simulink model "TestApp"  (R2014a)
settings: Solver=ode45  StartTime=0.0  StopTime=1  RelTol=1e-3
libraries: simulink x6, arduinolib x4
settings Model: Creator=beaverl  LastModifiedBy=beaverl

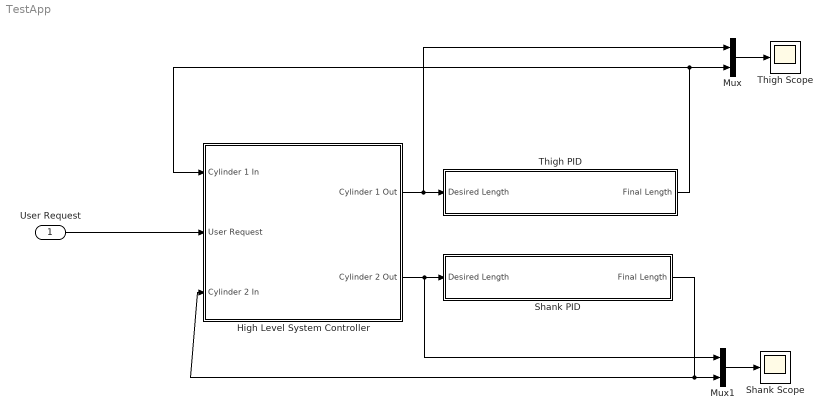
== system TestApp ==
  User Request : Inport
  High Level System Controller : Subsystem
  Mux : Mux  Inputs=2
  Mux1 : Mux  Inputs=2
  Shank PID : Subsystem
  Shank Scope : Scope
      settings: TimeRange=1  YMin=0  YMax=10
  Thigh PID : Subsystem
  Thigh Scope : Scope
      settings: TimeRange=1  YMin=0  YMax=10
  wires:
  Thigh PID/1(Final Length) -> High Level System Controller/1(Cylinder 1 In), Mux/2
  High Level System Controller/1(Cylinder 1 Out) -> Mux/1, Thigh PID/1(Desired Length)
  High Level System Controller/2(Cylinder 2 Out) -> Shank PID/1(Desired Length), Mux1/1
  Shank PID/1(Final Length) -> Mux1/2, High Level System Controller/3(Cylinder 2 In)
  Mux/1 -> Thigh Scope/1
  Mux1/1 -> Shank Scope/1
  User Request/1 -> High Level System Controller/2(User Request)

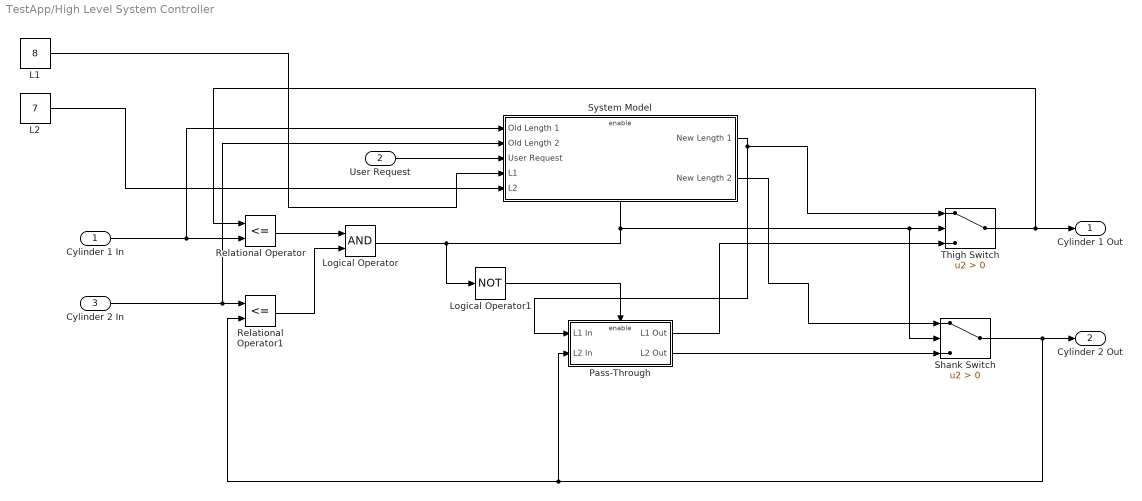
== system TestApp/High Level System Controller ==
  Cylinder 1 In : Inport
  User Request : Inport  Port=2
  Cylinder 2 In : Inport  Port=3
  L1 : Constant  Value=8
  L2 : Constant  Value=7
  Logical Operator : Logic  AllPortsSameDT=off  OutDataTypeStr=boolean
  Logical Operator1 : Logic  Operator=NOT  AllPortsSameDT=off  OutDataTypeStr=boolean
  Pass-Through : Subsystem  TreatAsAtomicUnit=on
  Relational Operator : RelationalOperator  Operator=<=  OutDataTypeStr=boolean
  Relational Operator1 : RelationalOperator  Operator=<=  OutDataTypeStr=boolean
  Shank Switch : Switch  Criteria=u2 > Threshold
  System Model : Subsystem
  Thigh Switch : Switch  Criteria=u2 > Threshold
  Cylinder 1 Out : Outport
  Cylinder 2 Out : Outport  Port=2
  wires:
  Cylinder 2 In/1 -> System Model/2(Old Length 2), Relational Operator1/1
  Cylinder 1 In/1 -> System Model/1(Old Length 1), Relational Operator/2
  System Model/1(New Length 1) -> Pass-Through/1(L1 In), Thigh Switch/1
  System Model/2(New Length 2) -> Shank Switch/1
  Relational Operator/1 -> Logical Operator/1
  Relational Operator1/1 -> Logical Operator/2
  Logical Operator/1 -> Logical Operator1/1, Shank Switch/2, Thigh Switch/2, System Model/Enable
  Logical Operator1/1 -> Pass-Through/Enable
  User Request/1 -> System Model/3(User Request)
  Thigh Switch/1 -> Relational Operator/1, Cylinder 1 Out/1
  Pass-Through/1(L1 Out) -> Thigh Switch/3
  Pass-Through/2(L2 Out) -> Shank Switch/3
  Shank Switch/1 -> Pass-Through/2(L2 In), Relational Operator1/2, Cylinder 2 Out/1
  L1/1 -> System Model/4(L1)
  L2/1 -> System Model/5(L2)

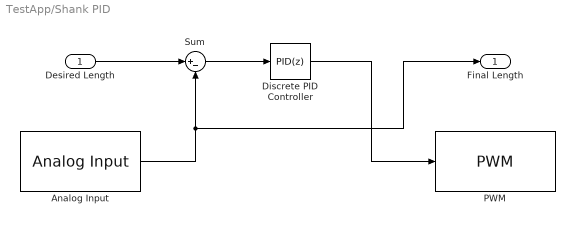
== system TestApp/Shank PID ==
  Desired Length : Inport
  Analog Input : arduinolib/Analog Input  pinNumber=6  sampleTime=-1
  Discrete PID Controller : simulink/Continuous/PID Controller  Controller=PID  TimeDomain=Discrete-time  SampleTime=-1  IntegratorMethod=Forward Euler  FilterMethod=Forward Euler  Form=Parallel  P=25  I=0.78  D=0  N=100  InitialConditionSource=internal  InitialConditionForIntegrator=0  InitialConditionForFilter=0  ExternalReset=none  LimitOutput=off  UpperSaturationLimit=inf  LowerSaturationLimit=-inf  LinearizeAsGain=off  AntiWindupMode=none  Kb=1  TrackingMode=off  Kt=1  PParamMin=[]  PParamMax=[]  IParamMin=[]  IParamMax=[]  DParamMin=[]  DParamMax=[]  NParamMin=[]  NParamMax=[]  KbParamMin=[]  KbParamMax=[]  KtParamMin=[]  KtParamMax=[]  POutMin=[]  POutMax=[]  IOutMin=[]  IOutMax=[]  DOutMin=[]  DOutMax=[]  NOutMin=[]  NOutMax=[]  KbOutMin=[]  KbOutMax=[]  KtOutMin=[]  KtOutMax=[]  IntegratorOutMin=[]  IntegratorOutMax=[]  FilterOutMin=[]  FilterOutMax=[]  SumOutMin=[]  SumOutMax=[]  SumI1OutMin=[]  SumI1OutMax=[]  SumI2OutMin=[]  SumI2OutMax=[]  SumI3OutMin=[]  SumI3OutMax=[]  SumDOutMin=[]  SumDOutMax=[]  SaturationOutMin=[]  SaturationOutMax=[]  IntegratorContinuousStateAttributes=''  IntegratorStateMustResolveToSignalObject=off  IntegratorRTWStateStorageClass=Auto  FilterContinuousStateAttributes=''  FilterStateMustResolveToSignalObject=off  FilterRTWStateStorageClass=Auto
  PWM : arduinolib/PWM  pinNumber=7
  Sum : Sum  Inputs=|+-
  Final Length : Outport
  wires:
  Desired Length/1 -> Sum/1
  Analog Input/1 -> Final Length/1, Sum/2
  Sum/1 -> Discrete PID Controller/1
  Discrete PID Controller/1 -> PWM/1

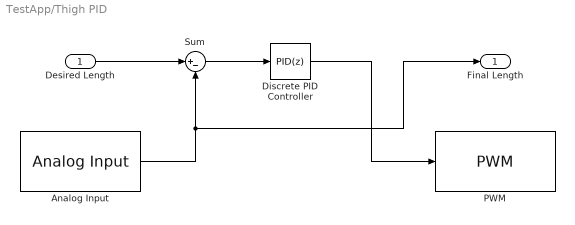
== system TestApp/Thigh PID ==
  Desired Length : Inport
  Analog Input : arduinolib/Analog Input  pinNumber=4  sampleTime=-1
  Discrete PID Controller : simulink/Continuous/PID Controller  Controller=PID  TimeDomain=Discrete-time  SampleTime=-1  IntegratorMethod=Forward Euler  FilterMethod=Forward Euler  Form=Parallel  P=25  I=0.78  D=0  N=100  InitialConditionSource=internal  InitialConditionForIntegrator=0  InitialConditionForFilter=0  ExternalReset=none  LimitOutput=off  UpperSaturationLimit=inf  LowerSaturationLimit=-inf  LinearizeAsGain=off  AntiWindupMode=none  Kb=1  TrackingMode=off  Kt=1  PParamMin=[]  PParamMax=[]  IParamMin=[]  IParamMax=[]  DParamMin=[]  DParamMax=[]  NParamMin=[]  NParamMax=[]  KbParamMin=[]  KbParamMax=[]  KtParamMin=[]  KtParamMax=[]  POutMin=[]  POutMax=[]  IOutMin=[]  IOutMax=[]  DOutMin=[]  DOutMax=[]  NOutMin=[]  NOutMax=[]  KbOutMin=[]  KbOutMax=[]  KtOutMin=[]  KtOutMax=[]  IntegratorOutMin=[]  IntegratorOutMax=[]  FilterOutMin=[]  FilterOutMax=[]  SumOutMin=[]  SumOutMax=[]  SumI1OutMin=[]  SumI1OutMax=[]  SumI2OutMin=[]  SumI2OutMax=[]  SumI3OutMin=[]  SumI3OutMax=[]  SumDOutMin=[]  SumDOutMax=[]  SaturationOutMin=[]  SaturationOutMax=[]  IntegratorContinuousStateAttributes=''  IntegratorStateMustResolveToSignalObject=off  IntegratorRTWStateStorageClass=Auto  FilterContinuousStateAttributes=''  FilterStateMustResolveToSignalObject=off  FilterRTWStateStorageClass=Auto
  PWM : arduinolib/PWM  pinNumber=5
  Sum : Sum  Inputs=|+-
  Final Length : Outport
  wires:
  Desired Length/1 -> Sum/1
  Analog Input/1 -> Final Length/1, Sum/2
  Sum/1 -> Discrete PID Controller/1
  Discrete PID Controller/1 -> PWM/1

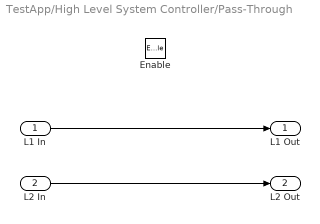
== system TestApp/High Level System Controller/Pass-Through ==
  L1 In : Inport
  L2 In : Inport  Port=2
  Enable : EnablePort
  L1 Out : Outport
  L2 Out : Outport  Port=2
  wires:
  L1 In/1 -> L1 Out/1
  L2 In/1 -> L2 Out/1

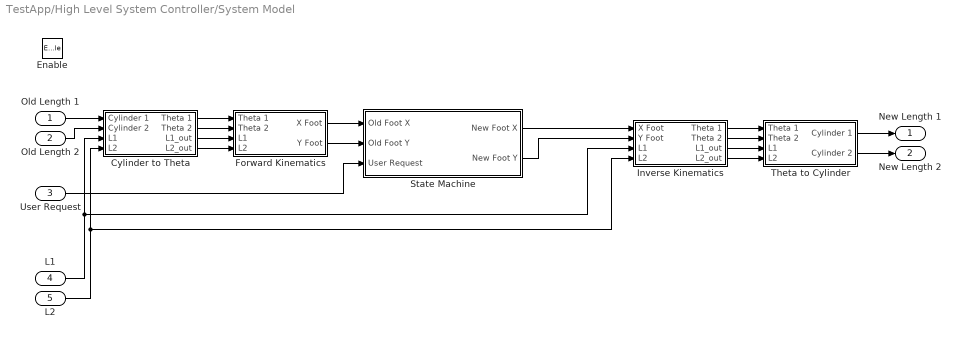
== system TestApp/High Level System Controller/System Model ==
  Old Length 1 : Inport
  Old Length 2 : Inport  Port=2
  User Request : Inport  Port=3
  L1 : Inport  Port=4
  L2 : Inport  Port=5
  Enable : EnablePort
  Cylinder to Theta : Subsystem
  Forward Kinematics : Subsystem
  Inverse Kinematics : Subsystem
  State Machine : Subsystem
  Theta to Cylinder : Subsystem
  New Length 1 : Outport
  New Length 2 : Outport  Port=2
  wires:
  Old Length 1/1 -> Cylinder to Theta/1(Cylinder 1)
  Old Length 2/1 -> Cylinder to Theta/2(Cylinder 2)
  Theta to Cylinder/2(Cylinder 2) -> New Length 2/1
  Theta to Cylinder/1(Cylinder 1) -> New Length 1/1
  Cylinder to Theta/1(Theta 1) -> Forward Kinematics/1(Theta 1)
  Cylinder to Theta/2(Theta 2) -> Forward Kinematics/2(Theta 2)
  Forward Kinematics/1(X Foot) -> State Machine/1(Old Foot X)
  Forward Kinematics/2(Y Foot) -> State Machine/2(Old Foot Y)
  State Machine/1(New Foot X) -> Inverse Kinematics/1(X Foot)
  State Machine/2(New Foot Y) -> Inverse Kinematics/2(Y Foot)
  Inverse Kinematics/1(Theta 1) -> Theta to Cylinder/1(Theta 1)
  Inverse Kinematics/2(Theta 2) -> Theta to Cylinder/2(Theta 2)
  User Request/1 -> State Machine/3(User Request)
  Cylinder to Theta/3(L1_out) -> Forward Kinematics/3(L1)
  Cylinder to Theta/4(L2_out) -> Forward Kinematics/4(L2)
  Inverse Kinematics/3(L1_out) -> Theta to Cylinder/3(L1)
  Inverse Kinematics/4(L2_out) -> Theta to Cylinder/4(L2)
  L1/1 -> Inverse Kinematics/3(L1), Cylinder to Theta/3(L1)
  L2/1 -> Inverse Kinematics/4(L2), Cylinder to Theta/4(L2)

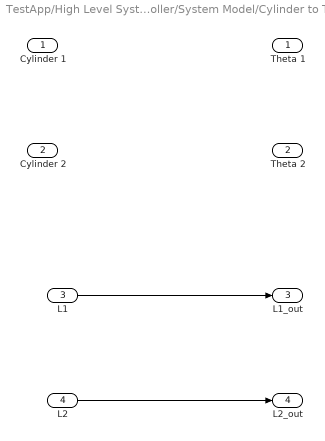
== system TestApp/High Level System Controller/System Model/Cylinder to Theta ==
  Cylinder 1 : Inport
  Cylinder 2 : Inport  Port=2
  L1 : Inport  Port=3
  L2 : Inport  Port=4
  Theta 1 : Outport
  Theta 2 : Outport  Port=2
  L1_out : Outport  Port=3
  L2_out : Outport  Port=4
  wires:
  L1/1 -> L1_out/1
  L2/1 -> L2_out/1

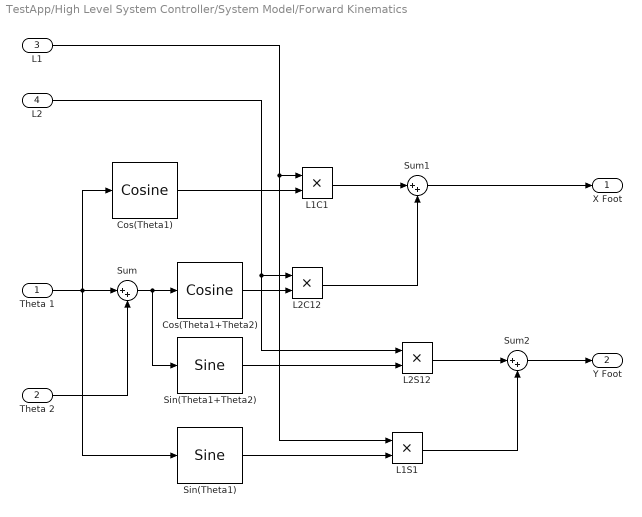
== system TestApp/High Level System Controller/System Model/Forward Kinematics ==
  Theta 1 : Inport
  Theta 2 : Inport  Port=2
  L1 : Inport  Port=3
  L2 : Inport  Port=4
  Cos(Theta1) : simulink/Lookup Tables/Cosine  Formula=cos(2*pi*u)  NumDataPoints=(2^5)+1  OutputWordLength=16  InternalRulePriority=Speed
  Cos(Theta1+Theta2) : simulink/Lookup Tables/Cosine  Formula=cos(2*pi*u)  NumDataPoints=(2^5)+1  OutputWordLength=16  InternalRulePriority=Speed
  L1C1 : Product
  L1S1 : Product
  L2C12 : Product
  L2S12 : Product
  Sin(Theta1) : simulink/Lookup Tables/Sine  Formula=sin(2*pi*u)  NumDataPoints=(2^5)+1  OutputWordLength=16  InternalRulePriority=Speed
  Sin(Theta1+Theta2) : simulink/Lookup Tables/Sine  Formula=sin(2*pi*u)  NumDataPoints=(2^5)+1  OutputWordLength=16  InternalRulePriority=Speed
  Sum : Sum  Inputs=|++
  Sum1 : Sum  Inputs=|++
  Sum2 : Sum  Inputs=|++
  X Foot : Outport
  Y Foot : Outport  Port=2
  wires:
  Theta 1/1 -> Cos(Theta1)/1, Sin(Theta1)/1, Sum/1
  Theta 2/1 -> Sum/2
  Sum/1 -> Sin(Theta1+Theta2)/1, Cos(Theta1+Theta2)/1
  Cos(Theta1)/1 -> L1C1/2
  L1C1/1 -> Sum1/1
  L2C12/1 -> Sum1/2
  Sum1/1 -> X Foot/1
  Cos(Theta1+Theta2)/1 -> L2C12/2
  L2S12/1 -> Sum2/1
  L1S1/1 -> Sum2/2
  Sin(Theta1)/1 -> L1S1/2
  Sin(Theta1+Theta2)/1 -> L2S12/2
  Sum2/1 -> Y Foot/1
  L1/1 -> L1S1/1, L1C1/1
  L2/1 -> L2S12/1, L2C12/1

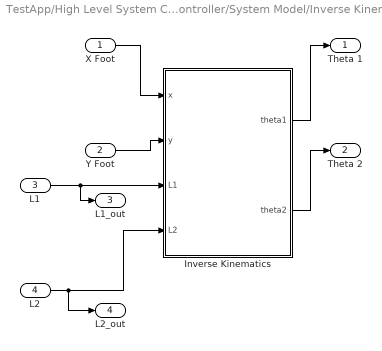
== system TestApp/High Level System Controller/System Model/Inverse Kinematics ==
  X Foot : Inport
  Y Foot : Inport  Port=2
  L1 : Inport  Port=3
  L2 : Inport  Port=4
  Inverse Kinematics : MATLAB Function  TreatAsAtomicUnit=on
  Theta 1 : Outport
  Theta 2 : Outport  Port=2
  L1_out : Outport  Port=3
  L2_out : Outport  Port=4
  wires:
  X Foot/1 -> Inverse Kinematics/1(x)
  Y Foot/1 -> Inverse Kinematics/2(y)
  Inverse Kinematics/1(theta1) -> Theta 1/1
  Inverse Kinematics/2(theta2) -> Theta 2/1
  L1/1 -> Inverse Kinematics/3(L1), L1_out/1
  L2/1 -> L2_out/1, Inverse Kinematics/4(L2)

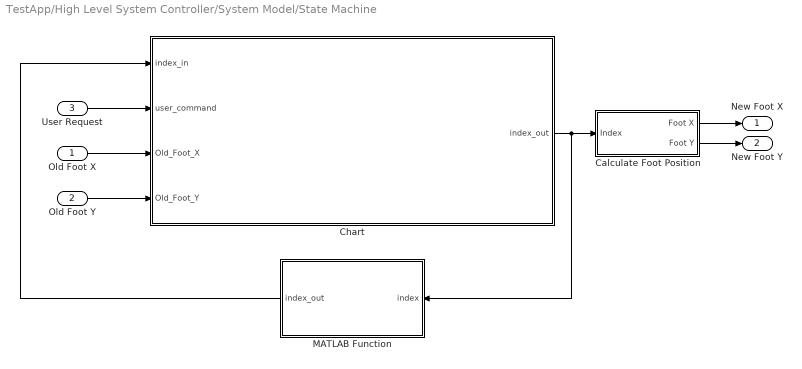
== system TestApp/High Level System Controller/System Model/State Machine ==
  Old Foot X : Inport
  Old Foot Y : Inport  Port=2
  User Request : Inport  Port=3
  Calculate Foot Position : Subsystem
  Chart : Stateflow chart  TreatAsAtomicUnit=on
  MATLAB Function : MATLAB Function  TreatAsAtomicUnit=on
  New Foot X : Outport
  New Foot Y : Outport  Port=2
  wires:
  User Request/1 -> Chart/2(user_command)
  Chart/1(index_out) -> MATLAB Function/1(index), Calculate Foot Position/1(Index)
  Calculate Foot Position/1(Foot X) -> New Foot X/1
  Calculate Foot Position/2(Foot Y) -> New Foot Y/1
  Old Foot Y/1 -> Chart/4(Old_Foot_Y)
  Old Foot X/1 -> Chart/3(Old_Foot_X)
  MATLAB Function/1(index_out) -> Chart/1(index_in)

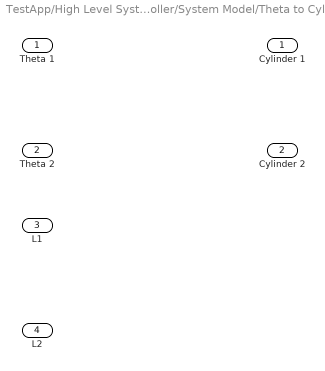
== system TestApp/High Level System Controller/System Model/Theta to Cylinder ==
  Theta 1 : Inport
  Theta 2 : Inport  Port=2
  L1 : Inport  Port=3
  L2 : Inport  Port=4
  Cylinder 1 : Outport
  Cylinder 2 : Outport  Port=2

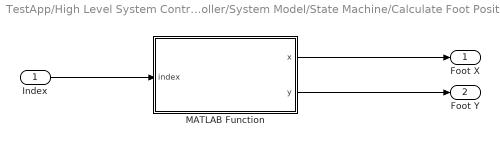
== system TestApp/High Level System Controller/System Model/State Machine/Calculate Foot Position ==
  Index : Inport
  MATLAB Function : MATLAB Function  TreatAsAtomicUnit=on
  Foot X : Outport
  Foot Y : Outport  Port=2
  wires:
  MATLAB Function/1(x) -> Foot X/1
  MATLAB Function/2(y) -> Foot Y/1
  Index/1 -> MATLAB Function/1(index)

== matlab function TestApp/High Level System Controller/System Model/State Machine/Calculate Foot Position/MATLAB Function ==
  data: x output; index input; y output
function [x, y] = LookupTable(index)
%#codegen
Array = [1:5, 5:-1:1; 5:-1:1, 1:5];

y = Array(index);
x = Array(index);

== matlab function TestApp/High Level System Controller/System Model/Inverse Kinematics/Inverse Kinematics ==
  data: x input; theta1 output; theta2 output; y input; L1 input; L2 input
function [theta1, theta2] = fcn(x, y, L1, L2)
%"max(..., 0)" is used to ensure the robot stays within its operational bounds
num = max((L1+L2)^2 - (x^2 + y^2), 0);
den = max((x^2 + y^2) - (L1-L2)^2, 0);
theta2 = -2*atan2(sqrt(num),sqrt(den));
num = y*(L1+L2*cos(theta2)) - L2*x*sin(theta2);
den = x*(L1+L2*cos(theta2)) + L2*y*sin(theta2);
theta1 = atan2(num,den)*180/pi;
theta2 = theta2*180/pi;
end

== stateflow chart TestApp/High Level System Controller/System Model/State Machine/Chart ==
  state Idle
    entry: index_out = index_in;
  state Forward
    entry: index_out = index_in + 1;
  state Reverse
    entry: index_out = index_in - 1;
  Reverse -> Idle : [user_command ~= -1]
  (default) -> Idle
  Idle -> Forward [order 1] : [user_command == 1]
  Forward -> Idle : [user_command ~= 1]
  Idle -> Reverse [order 2] : [user_command == -1]
  data: index_in input int32; user_command input; index_out output; Old_Foot_X input; Old_Foot_Y input

== matlab function TestApp/High Level System Controller/System Model/State Machine/MATLAB Function ==
  data: index_out output; index input
function index_out = ClampIndex(index)
%#codegen
if index > 10
    index = 1;
end
if index < 1
    index = 10;
end
index_out = index;
